simulink model "quarter_car_model_advanced"  (R2023b)
settings: Solver=VariableStepAuto  StartTime=0.0  StopTime=100  RelTol=1e-3
values from neighbouring files (symbols this model uses):
  c1 = 12    [data_small_racing_vehicle.m]
  k1 = 23    [data_small_racing_vehicle.m]
  k2 = 700    [data_small_racing_vehicle.m]
  mc = 60    [data_small_racing_vehicle.m]
  ms = 12    [data_small_racing_vehicle.m]
settings Model: Creator=NITRO  LastModifiedBy=NITRO

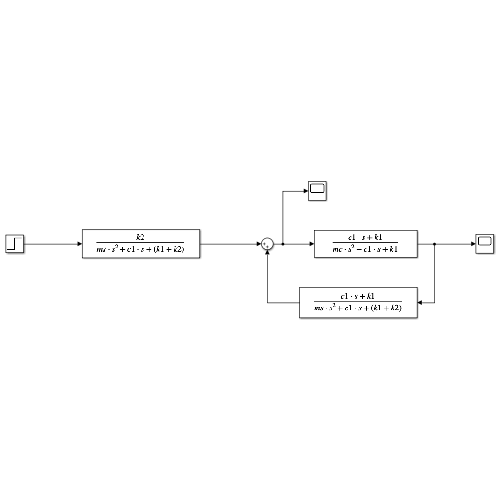
[thumbnail: Simulink's stored preview of the top-level diagram]
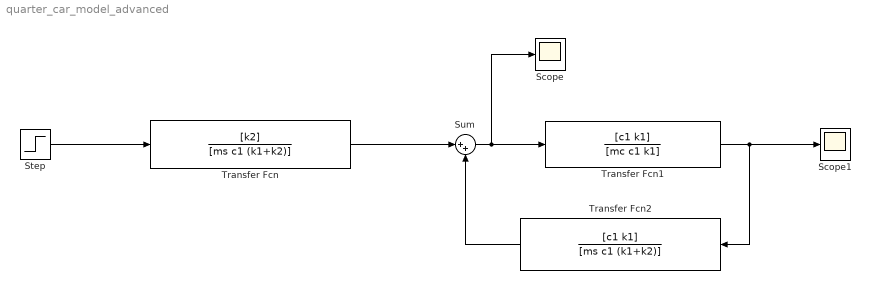
== system quarter_car_model_advanced ==
  Scope : Scope
  Scope1 : Scope
  Step : Step  After=30  SampleTime=0
  Sum : Sum  Inputs=|++
  Transfer Fcn : TransferFcn  Numerator=[k2]  Denominator=[ms c1 (k1+k2)]
  Transfer Fcn1 : TransferFcn  Numerator=[c1 k1]  Denominator=[mc c1 k1]
  Transfer Fcn2 : TransferFcn  Numerator=[c1 k1]  Denominator=[ms c1 (k1+k2)]
  wires:
  Transfer Fcn/1 -> Sum/1
  Sum/1 -> Scope/1, Transfer Fcn1/1
  Transfer Fcn2/1 -> Sum/2
  Step/1 -> Transfer Fcn/1
  Transfer Fcn1/1 -> Transfer Fcn2/1, Scope1/1
